simulink model "Modell_13_3"  (R2018a)
settings: Solver=VariableStepAuto  StartTime=0.0  StopTime=10.0  RelTol=1e-3
InitFcn:
  | init_13_3
values from neighbouring files (symbols this model uses):
  a = 1    [init_13_1.m]    (also in init_13_3.m)
  b = 1    [init_13_1.m]    (also in init_13_3.m)
  c = 1    [init_13_1.m]    (also in init_13_3.m)
  kS = 0.2    [init_13_1.m]    (also in init_13_3.m)
  kT = 1    [init_13_1.m]    (also in init_13_3.m)
  S01 = 0.2    [init_13_1.m]    (also in init_13_3.m)
  S02 = 2    [init_13_1.m]    (also in init_13_3.m)
  S1 = 0.4    [init_13_1.m]    (also in init_13_3.m)
  S2 = 1.6    [init_13_1.m]    (also in init_13_3.m)
  T01 = 3    [init_13_1.m]    (also in init_13_3.m)
  T02 = 0.5    [init_13_1.m]    (also in init_13_3.m)
  T1 = 1.2    [init_13_1.m]    (also in init_13_3.m)
  T2 = 1    [init_13_1.m]    (also in init_13_3.m)
settings Model: Creator=Uni  LastModifiedBy=Uni

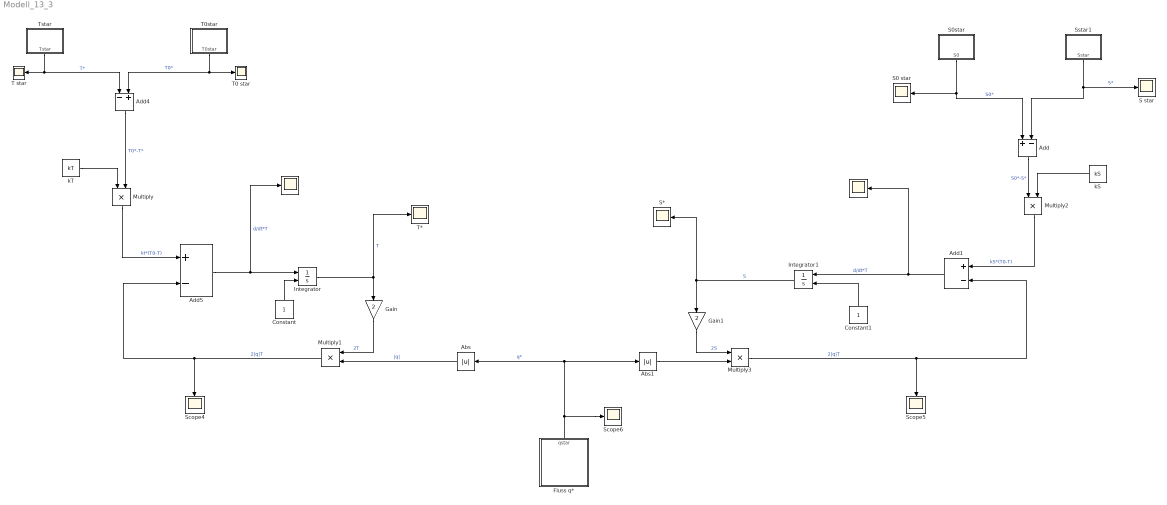
== system Modell_13_3 ==
  " " : Scope
  "  " : Scope
  Abs : Abs
  Abs1 : Abs
  Add : Sum  Inputs=+-
  Add1 : Sum  Inputs=+-
  Add4 : Sum  Inputs=-+
  Add5 : Sum  Inputs=+-
  Constant : Constant
  Constant1 : Constant
  Fluss q* : Subsystem
  Gain : Gain  Gain=2
  Gain1 : Gain  Gain=2
  Integrator : Integrator  InitialConditionSource=external
  Integrator1 : Integrator  InitialConditionSource=external
  Multiply{,1..3} (4 alike) : Product
  S star : Scope
  "S* " : Scope
  S0 star : Scope
  S0star : Subsystem
  Scope4 : Scope
  Scope5 : Scope
  Scope6 : Scope
  Sstar1 : Subsystem
  T star : Scope
  "T* " : Scope
  T0 star : Scope
  T0star : Subsystem
  Tstar : Subsystem
  kS : Constant  Value=kS
  kT : Constant  Value=kT
  wires:
  Add4/1 -> Multiply/2  "T0*-T*"
  kT/1 -> Multiply/1
  Multiply/1 -> Add5/1  "kt*(T0-T)"
  Constant/1 -> Integrator/2
  Add5/1 -> " "/1, Integrator/1  "d/dt*T"
  Integrator/1 -> Gain/1, "T* "/1  "T"
  Gain/1 -> Multiply1/1  "2T"
  Multiply1/1 -> Add5/2, Scope4/1  "2|q|T"
  Abs/1 -> Multiply1/2  "|q|"
  T0star/1(T0star) -> T0 star/1, Add4/2  "T0*"
  Tstar/1(Tstar) -> Add4/1, T star/1  "T*"
  Fluss q*/1(qstar) -> Scope6/1, Abs1/1, Abs/1  "q*"
  Sstar1/1(Sstar) -> Add/2, S star/1  "S*"
  S0star/1(S0) -> S0 star/1, Add/1  "S0*"
  Add/1 -> Multiply2/1  "S0*-S*"
  kS/1 -> Multiply2/2
  Multiply2/1 -> Add1/1  "kS*(T0-T)"
  Add1/1 -> Integrator1/1, "  "/1  "d/dt*T"
  Constant1/1 -> Integrator1/2
  Integrator1/1 -> Gain1/1, "S* "/1  "S"
  Gain1/1 -> Multiply3/1  "2S"
  Abs1/1 -> Multiply3/2
  Multiply3/1 -> Scope5/1, Add1/2  "2|q|T"

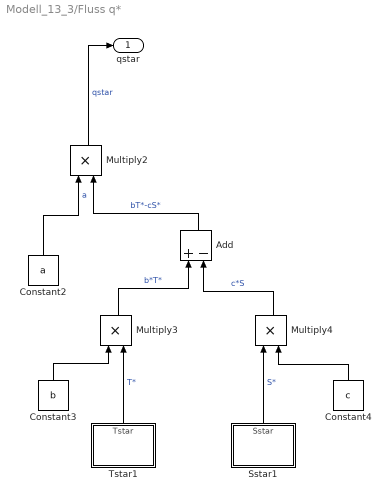
== system Modell_13_3/Fluss q* ==
  Add : Sum  Inputs=+-
  Constant2 : Constant  Value=a
  Constant3 : Constant  Value=b
  Constant4 : Constant  Value=c
  Multiply2 : Product
  Multiply3 : Product
  Multiply4 : Product
  Sstar1 : Subsystem
  Tstar1 : Subsystem
  qstar : Outport
  wires:
  Multiply2/1 -> qstar/1  "qstar"
  Multiply4/1 -> Add/2  "c*S"
  Constant3/1 -> Multiply3/1
  Tstar1/1(Tstar) -> Multiply3/2  "T*"
  Multiply3/1 -> Add/1  "b*T*"
  Add/1 -> Multiply2/2  "bT*-cS*"
  Sstar1/1(Sstar) -> Multiply4/1  "S*"
  Constant2/1 -> Multiply2/1  "a"
  Constant4/1 -> Multiply4/2

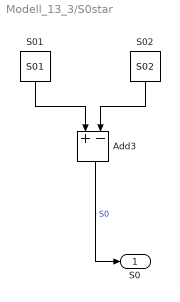
== system Modell_13_3/S0star ==
  Add3 : Sum  Inputs=+-
  S01 : Constant  Value=S01
  S02 : Constant  Value=S02
  S0 : Outport
  wires:
  Add3/1 -> S0/1  "S0"
  S02/1 -> Add3/2
  S01/1 -> Add3/1

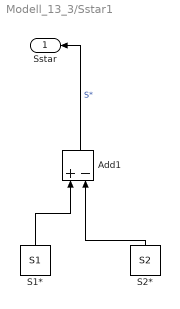
== system Modell_13_3/Sstar1 ==
  Add1 : Sum  Inputs=+-
  S1* : Constant  Value=S1
  S2* : Constant  Value=S2
  Sstar : Outport
  wires:
  S1*/1 -> Add1/1
  S2*/1 -> Add1/2
  Add1/1 -> Sstar/1  "S*"

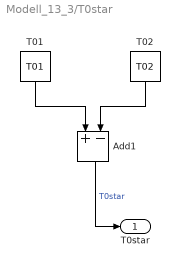
== system Modell_13_3/T0star ==
  Add1 : Sum  Inputs=+-
  T01 : Constant  Value=T01
  T02 : Constant  Value=T02
  T0star : Outport
  wires:
  T01/1 -> Add1/1
  Add1/1 -> T0star/1  "T0star"
  T02/1 -> Add1/2

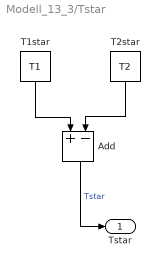
== system Modell_13_3/Tstar ==
  Add : Sum  Inputs=+-
  T1star : Constant  Value=T1
  T2star : Constant  Value=T2
  Tstar : Outport
  wires:
  T1star/1 -> Add/1
  T2star/1 -> Add/2
  Add/1 -> Tstar/1  "Tstar"

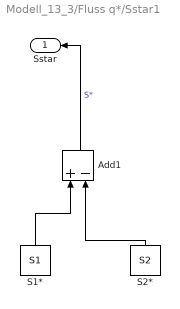
== system Modell_13_3/Fluss q*/Sstar1 ==
  Add1 : Sum  Inputs=+-
  S1* : Constant  Value=S1
  S2* : Constant  Value=S2
  Sstar : Outport
  wires:
  S1*/1 -> Add1/1
  S2*/1 -> Add1/2
  Add1/1 -> Sstar/1  "S*"

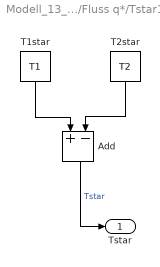
== system Modell_13_3/Fluss q*/Tstar1 ==
  Add : Sum  Inputs=+-
  T1star : Constant  Value=T1
  T2star : Constant  Value=T2
  Tstar : Outport
  wires:
  T1star/1 -> Add/1
  T2star/1 -> Add/2
  Add/1 -> Tstar/1  "Tstar"
